simulink model "DFADAS2_SenFus_v1_201204RC_training_210115"  (R2018b)
settings: Solver=FixedStepDiscrete  StartTime=0.0  StopTime=inf  FixedStep=0.002  RelTol=1e-3  EnableMultiTasking=on
PreLoadFcn:
  | RTWConfigurationCB('preloadfcn', bdroot);
libraries: canmsglib x108, simulink x48, canfdmsglib x12
(part 11 of 28)

== system DFADAS2_SenFus_v1_201204RC_training_210115/Signal Input (Input)/Signal Input (10ms) (Input10)/VehInfo/Function Keys State Receive and Processing (FKeyStRx)/Key Enable CAN Frame PreProcess (KeyEnaCANFrmPPrcs) ==
  Bus Creator : BusCreator  Inputs=2
  CAN Diagnosis (CANDia) : Subsystem  Commented=on
  CAN Receive Sample Time : Constant  Value=0.02  OutDataTypeStr=single  SampleTime=-1
  CAN Unpack : canmsglib/CAN Unpack  CANdbFile=F:\LD\3_simulinkModel_13b\TJAHWA\ADAS_D53_PSA1CAN_LiPiao_DLC.dbc  MsgList=GW_309_PSA1  MsgName=GW_309_PSA1  MsgIDType=Standard (11-bit identifier)  MsgIdentifier=777  MsgLength=8  SignalInfo=GW_SCC_LeftSteeringWheelSwitch$0$8$2$2$1$0$1$0$-Inf$Inf$#GW_SCC_RightSteeringWheelSwitch$8$8$2$2$1$0$1$0$-Inf$Inf$#  NSignals=2  IDPort=off  TimestampPort=off  ErrorPort=off  RemotePort=off  LengthPort=off  StatusPort=off  StartBits=str2num('[int32(0);int32(8)]')  SignalSizes=str2num('[int32(8);int32(8)]')  ByteOrders=str2num('[int32(2);int32(2)]')  DataTypes=str2num('[int32(2);int32(2)]')  MultiplexTypes=str2num('[int32(1);int32(1)]')  MultiplexValues=str2num('[double(0);double(0)]')  Factors=str2num('[double(1);double(1)]')  Offsets=str2num('[double(0);double(0)]')  Minimums=str2num('[double(-Inf);double(-Inf)]')  Maximums=str2num('[double(Inf);double(Inf)]')  ApplyMinMax=off
      settings: SourceProductName=Simulink Real-Time  SourceProductBaseCode=XP  DataFormat=CANdb specified signals
  Data Type Conversion1 : DataTypeConversion  OutDataTypeStr=single
  Data Type Conversion3 : DataTypeConversion  OutDataTypeStr=single
  Rate Transition1 : RateTransition  OutPortSampleTime=0.01
  Rate Transition4 : RateTransition  OutPortSampleTime=0.01
  S-Function1 : S-Function  FunctionName=NSTC297CANReceiveBlkLib  Parameters=|  SFunctionDeploymentMode=off  EnableBusSupport=off  mask(NSTC297 CAN Receive){Ns_DeviceID=ADAS Control Unit Gen2, Ns_ChannelNum=4, Ns_FrameID=777, Ns_IsVirtualFrame=off, Ns_RoleInVirtualFrame=Header Frame, Ns_HeaderFrameID=0, Ns_VirtualFrameStatusFlg=off, Ns_IncompleteFrameCntFlg=off, Ns_OverflowCntFlg=off, Ns_FrameBufferSize=1, Ns_SampleTime=0.01}
      | uint16(Ns_DeviceID),
      | uint16(Ns_ChannelNum),
      | uint32(Ns_FrameID),
      | uint8(Ns_IsVirtualFrame),
      | uint16(Ns_RoleInVirtualFrame),
      | uint32(Ns_HeaderFrameID),
      | uint8(Ns_VirtualFrameStatusFlg),
      | uint8(Ns_IncompleteFrameCntFlg),
      | uint8(Ns_OverflowCntFlg),
      | uint16(Ns_FrameBufferSize),
      | double(Ns_SampleTime)
      mask prompts: Ns_DeviceID "Device:"; Ns_ChannelNum "Channel number:"; Ns_FrameID "Frame ID:"; Ns_IsVirtualFrame "Belong to a virtual frame"; Ns_RoleInVirtualFrame "Position in virtual frame:"; Ns_HeaderFrameID "Header frame ID:"; Ns_VirtualFrameStatusFlg "Current virtural frame status output"; Ns_IncompleteFrameCntFlg "Incomplete virtual frame count output"; Ns_OverflowCntFlg "Overflow count output"; Ns_FrameBufferSize "Frame buffer size:"; Ns_SampleTime "Sample time:"
      mask init:
      | NSTC297CANReceive_callback('portlabels');
      mask TypeOptions Ns_DeviceID: General Control Unit Gen2 | ADAS Control Unit Gen2
      mask TypeOptions Ns_ChannelNum: 0 | 1 | 2 | 3 | 4 | 5
      mask Callback Ns_IsVirtualFrame: NSTC297CANReceive_callback('Belong to a virtual frame');
      mask TypeOptions Ns_RoleInVirtualFrame: Header Frame | Data Frame | Trailer Frame
      mask Callback Ns_RoleInVirtualFrame: NSTC297CANReceive_callback('Position in virtual frame');
      mask Display: color('blue');text(0.02,0.9,'NovSteeds TC297','horizontalAlignment','left');color('blue');text(0.5,0.7,'CAN Receive','horizontalAlignment','center');color('black');text(0.5,0.6,'Channel: 4','horizontalAlignment','center');text(0.5,0.5,'ID: 777','horizontalAlignment','center');text(0.5,0.4,'Virtual Frame: No','horizontalAlignment','center');port_label('output',1, 'RemainderCnt');port_label('output',2, 'Msg');
  Time Limit : Constant  OutDataTypeStr=single  SampleTime=-1
  IC_RightSteeringWheelSwitchSig : Outport
  wires:
  Rate Transition4/1 -> Data Type Conversion3/1
  CAN Unpack/1 -> Rate Transition4/1
  CAN Receive Sample Time/1 -> CAN Diagnosis (CANDia)/1(CANDia_tiCANRxSmplT)
  Time Limit/1 -> CAN Diagnosis (CANDia)/2(CANDia_tiTLim)
  S-Function1/1 -> CAN Diagnosis (CANDia)/3(CANDia_cfNewFlg)
  S-Function1/2 -> CAN Unpack/1, CAN Diagnosis (CANDia)/4(CANDia_regCANMsg)
  Rate Transition1/1 -> Data Type Conversion1/1
  CAN Unpack/2 -> Rate Transition1/1
  Data Type Conversion3/1 -> Bus Creator/1  "GW_LeftSteeringWheelS"
  Data Type Conversion1/1 -> Bus Creator/2  "GW_RightSteeringWheelS"
  Bus Creator/1 -> IC_RightSteeringWheelSwitchSig/1

== system DFADAS2_SenFus_v1_201204RC_training_210115/Signal Input (Input)/Signal Input (10ms) (Input10)/VehInfo/MP5 Signal Receive (MP5Rx)1/CAN Diagnosis (CANDia) ==
  CANDia_tiCANRxSmplT : Inport
  CANDia_tiTLim : Inport  Port=2
  CANDia_cfNewFlg : Inport  Port=3
  CANDia_regCANMsg : Inport  Port=4
  CANDia_ctRllCnt : Inport  Port=5
  Break State Diagnosis (BreStDia) : Subsystem
  CAN Frame DTC Generator (CANFrmDTCGtr) : Subsystem
  CheckSum Diagnosis (ChkSumDia) : Subsystem
  RollingCounter Diagnosis (RllCntDia) : Subsystem
  wires:
  CANDia_regCANMsg/1 -> CheckSum Diagnosis (ChkSumDia)/1(ChkSumDia_regCANMsgPrev)
  CANDia_ctRllCnt/1 -> RollingCounter Diagnosis (RllCntDia)/1(RllCntChk_ctRollingCounter)
  RollingCounter Diagnosis (RllCntDia)/1(RllCntChk_efErrorFlag) -> CAN Frame DTC Generator (CANFrmDTCGtr)/3(CANFrmDTCGtr_efRllCntDiaErrFlg)
  Break State Diagnosis (BreStDia)/1(BreStDia_efErrFlg) -> CAN Frame DTC Generator (CANFrmDTCGtr)/1(CANFrmDTCGtr_efBreStDiaErrFlg)
  CheckSum Diagnosis (ChkSumDia)/1(ChkSumDia_efErrFlg) -> CAN Frame DTC Generator (CANFrmDTCGtr)/2(CANFrmDTCGtr_efChkSumDiaErrFlg)
  CANDia_cfNewFlg/1 -> Break State Diagnosis (BreStDia)/3(BreStDia_cfCANRxNewFlg)
  CANDia_tiTLim/1 -> Break State Diagnosis (BreStDia)/2(BreStDia_tiTLim)
  CANDia_tiCANRxSmplT/1 -> Break State Diagnosis (BreStDia)/1(BreStDia_tiCANRxSmplT)

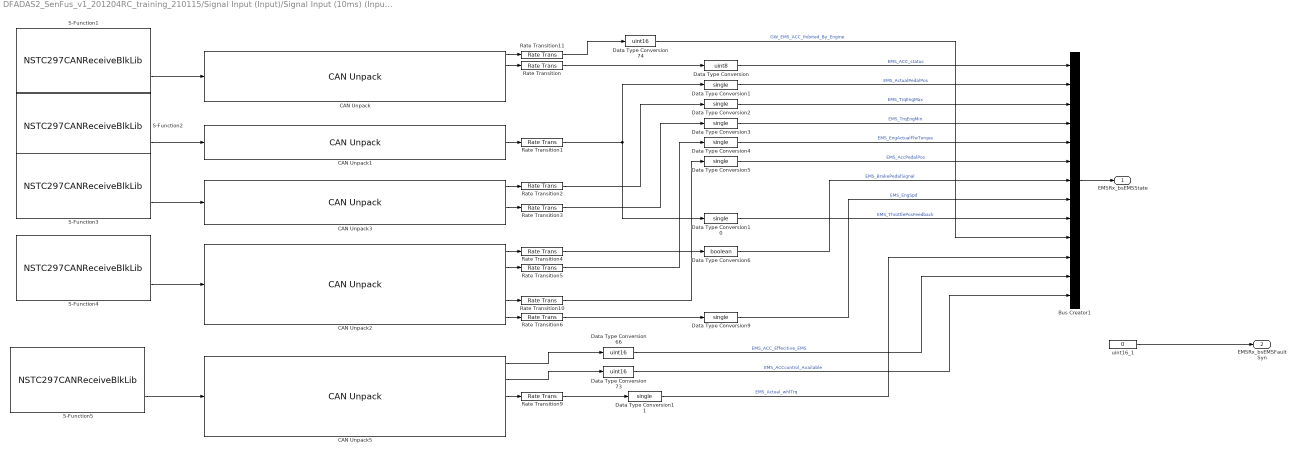
== system DFADAS2_SenFus_v1_201204RC_training_210115/Signal Input (Input)/Signal Input (10ms) (Input10)/VehInfo/Powertrain State Receive and Processing (PTRx)/EMS State Receive and Processing (EMSRx) ==
  Bus Creator1 : BusCreator  Inputs=13
  CAN Unpack : canmsglib/CAN Unpack  CANdbFile=F:\ADAS_File\ACC_AEB_D53_20190520\ADAS_ECU_PSA1_CAN_V2_v20190520.dbc  MsgList=GW_2D8_PSA1  MsgName=GW_2D8_PSA1  MsgIDType=Standard (11-bit identifier)  MsgIdentifier=728  MsgLength=7  SignalInfo=GW_EMS_ACC_Ihibited_By_Engine$52$1$2$2$1$0$1$0$0$1$#GW_EMS_EMS_Status_ACC$16$3$2$2$1$0$1$0$0$7$#GW_EMS_Pot_WhlTrq_Max$37$11$2$2$1$0$8$-4000$-4000$11000$#GW_EMS_Pot_WhlTrq_Min$53$11$2$2$1$0$8$-4000$-4000$11000$#GW_EMS_Pot_WhlTrq_Request$19$13$2$2$1$0$2$-4000$-4000$11000$#  NSignals=5  IDPort=off  TimestampPort=off  ErrorPort=off  RemotePort=off  LengthPort=off  StatusPort=off  StartBits=str2num('[int32(52);int32(16);int32(37);int32(53);int32(19)]')  SignalSizes=str2num('[int32(1);int32(3);int32(11);int32(11);int32(13)]')  ByteOrders=str2num('[int32(2);int32(2);int32(2);int32(2);int32(2)]')  DataTypes=str2num('[int32(2);int32(2);int32(2);int32(2);int32(2)]')  MultiplexTypes=str2num('[int32(1);int32(1);int32(1);int32(1);int32(1)]')  MultiplexValues=str2num('[double(0);double(0);double(0);double(0);double(0)]')  Factors=str2num('[double(1);double(1);double(8);double(8);double(2)]')  Offsets=str2num('[double(0);double(0);double(-4000);double(-4000);double(-4000)]')  Minimums=str2num('[double(0);double(0);double(-4000);double(-4000);double(-4000)]')  Maximums=str2num('[double(1);double(7);double(11000);double(11000);double(11000)]')  ApplyMinMax=off
      settings: SourceProductName=Simulink Real-Time  SourceProductBaseCode=XP  DataFormat=CANdb specified signals
  CAN Unpack1 : canmsglib/CAN Unpack  CANdbFile=F:\ADAS_File\ACC_AEB_D53_20190520\ADAS_ECU_PSA1_CAN_V2_v20190520.dbc  MsgList=GW_228_PSA1  MsgName=GW_228_PSA1  MsgIDType=Standard (11-bit identifier)  MsgIdentifier=552  MsgLength=8  SignalInfo=EMS_Acceleration_pedal_position$16$8$2$2$1$0$5.000000e-01$0$0$100$#  NSignals=1  IDPort=off  TimestampPort=off  ErrorPort=off  RemotePort=off  LengthPort=off  StatusPort=off  StartBits=str2num('[int32(16)]')  SignalSizes=str2num('[int32(8)]')  ByteOrders=str2num('[int32(2)]')  DataTypes=str2num('[int32(2)]')  MultiplexTypes=str2num('[int32(1)]')  MultiplexValues=str2num('[double(0)]')  Factors=str2num('[double(5.000000e-01)]')  Offsets=str2num('[double(0)]')  Minimums=str2num('[double(0)]')  Maximums=str2num('[double(100)]')  ApplyMinMax=off
      settings: SourceProductName=Simulink Real-Time  SourceProductBaseCode=XP  DataFormat=CANdb specified signals
  CAN Unpack2 : canmsglib/CAN Unpack  CANdbFile=F:\ADAS_File\ACC_AEB_D53_20190520\ADAS_ECU_PSA1_CAN_V2_v20190520.dbc  MsgList=GW_208_PSA1  MsgName=GW_208_PSA1  MsgIDType=Standard (11-bit identifier)  MsgIdentifier=520  MsgLength=8  SignalInfo=Brake_secondary_contact$33$1$2$2$1$0$1$0$-Inf$Inf$#EMS_Actual_torque$16$8$2$2$1$0$2$-100$-100$408$#EMS_DiagMuxOn$38$1$2$2$1$0$1$0$-Inf$Inf$#EMS_Driver_request$24$8$2$2$1$0$5.000000e-01$0$0$100$#EMS_Engine_RPM$8$16$2$2$1$0$1.250000e-01$0$0$8.191750e+03$#  NSignals=5  IDPort=off  TimestampPort=off  ErrorPort=off  RemotePort=off  LengthPort=off  StatusPort=off  StartBits=str2num('[int32(33);int32(16);int32(38);int32(24);int32(8)]')  SignalSizes=str2num('[int32(1);int32(8);int32(1);int32(8);int32(16)]')  ByteOrders=str2num('[int32(2);int32(2);int32(2);int32(2);int32(2)]')  DataTypes=str2num('[int32(2);int32(2);int32(2);int32(2);int32(2)]')  MultiplexTypes=str2num('[int32(1);int32(1);int32(1);int32(1);int32(1)]')  MultiplexValues=str2num('[double(0);double(0);double(0);double(0);double(0)]')  Factors=str2num('[double(1);double(2);double(1);double(5.000000e-01);double(1.250000e-01)]')  Offsets=str2num('[double(0);double(-100);double(0);double(0);double(0)]')  Minimums=str2num('[double(-Inf);double(-100);double(-Inf);double(0);double(0)]')  Maximums=str2num('[double(Inf);double(408);double(Inf);double(100);double(8.191750e+03)]')  ApplyMinMax=off
      settings: SourceProductName=Simulink Real-Time  SourceProductBaseCode=XP  DataFormat=CANdb specified signals
  CAN Unpack3 : canmsglib/CAN Unpack  CANdbFile=F:\ADAS_File\ACC_AEB_D53_20190520\ADAS_ECU_PSA1_CAN_V2_v20190520.dbc  MsgList=GW_2F8_PSA1  MsgName=GW_2F8_PSA1  MsgIDType=Standard (11-bit identifier)  MsgIdentifier=760  MsgLength=7  SignalInfo=EMS_WhlTrq_max$19$13$2$2$1$0$2$-4000$-4000$11000$#EMS_WhlTrq_max_offset$24$11$2$2$1$0$2$0$0$4000$#EMS_WhlTrq_min$43$13$2$2$1$0$2$-4000$-4000$11000$#EMS_WhlTrq_min_offset$48$11$2$2$1$0$2$0$0$4000$#  NSignals=4  IDPort=off  TimestampPort=off  ErrorPort=off  RemotePort=off  LengthPort=off  StatusPort=off  StartBits=str2num('[int32(19);int32(24);int32(43);int32(48)]')  SignalSizes=str2num('[int32(13);int32(11);int32(13);int32(11)]')  ByteOrders=str2num('[int32(2);int32(2);int32(2);int32(2)]')  DataTypes=str2num('[int32(2);int32(2);int32(2);int32(2)]')  MultiplexTypes=str2num('[int32(1);int32(1);int32(1);int32(1)]')  MultiplexValues=str2num('[double(0);double(0);double(0);double(0)]')  Factors=str2num('[double(2);double(2);double(2);double(2)]')  Offsets=str2num('[double(-4000);double(0);double(-4000);double(0)]')  Minimums=str2num('[double(-4000);double(0);double(-4000);double(0)]')  Maximums=str2num('[double(11000);double(4000);double(11000);double(4000)]')  ApplyMinMax=off
      settings: SourceProductName=Simulink Real-Time  SourceProductBaseCode=XP  DataFormat=CANdb specified signals
  CAN Unpack5 : canmsglib/CAN Unpack  CANdbFile=F:\ADAS_File\ACC_AEB_D53_20190520\ADAS_ECU_PSA1_CAN_V2_v20190520.dbc  MsgList=GW_318_PSA1  MsgName=GW_318_PSA1  MsgIDType=Standard (11-bit identifier)  MsgIdentifier=792  MsgLength=5  SignalInfo=EMS_ACC_Effecitive_EMS$33$1$2$2$1$0$1$0$0$1$#EMS_ACCcontrol_Available$17$1$2$2$1$0$1$0$0$1$#EMS_Actual_whlTrq$34$14$2$2$1$0$1$-4000$-4000$11000$#EMS_Driver_wheel_torque$18$14$2$2$1$0$1$-4000$-4000$11000$#EMS_GearBox_ACCcontrol_Available$16$1$2$2$1$0$1$0$0$1$#  NSignals=5  IDPort=off  TimestampPort=off  ErrorPort=off  RemotePort=off  LengthPort=off  StatusPort=off  StartBits=str2num('[int32(33);int32(17);int32(34);int32(18);int32(16)]')  SignalSizes=str2num('[int32(1);int32(1);int32(14);int32(14);int32(1)]')  ByteOrders=str2num('[int32(2);int32(2);int32(2);int32(2);int32(2)]')  DataTypes=str2num('[int32(2);int32(2);int32(2);int32(2);int32(2)]')  MultiplexTypes=str2num('[int32(1);int32(1);int32(1);int32(1);int32(1)]')  MultiplexValues=str2num('[double(0);double(0);double(0);double(0);double(0)]')  Factors=str2num('[double(1);double(1);double(1);double(1);double(1)]')  Offsets=str2num('[double(0);double(0);double(-4000);double(-4000);double(0)]')  Minimums=str2num('[double(0);double(0);double(-4000);double(-4000);double(0)]')  Maximums=str2num('[double(1);double(1);double(11000);double(11000);double(1)]')  ApplyMinMax=off
      settings: SourceProductName=Simulink Real-Time  SourceProductBaseCode=XP  DataFormat=CANdb specified signals
  Data Type Conversion : DataTypeConversion  OutDataTypeStr=uint8
  Data Type Conversion{1..5,9..11} (8 alike) : DataTypeConversion  OutDataTypeStr=single
  Data Type Conversion6 : DataTypeConversion  OutDataTypeStr=boolean
  Data Type Conversion66 : DataTypeConversion  OutDataTypeStr=uint16
  Data Type Conversion73 : DataTypeConversion  OutDataTypeStr=uint16
  Data Type Conversion74 : DataTypeConversion  OutDataTypeStr=uint16
  Rate Transition{,1..6,9..11} (10 alike) : RateTransition  OutPortSampleTime=0.01
  S-Function1 : S-Function  FunctionName=NSTC297CANReceiveBlkLib  Parameters=|  SFunctionDeploymentMode=off  EnableBusSupport=off  mask(NSTC297 CAN Receive){Ns_DeviceID=ADAS Control Unit Gen2, Ns_ChannelNum=4, Ns_FrameID=728, Ns_IsVirtualFrame=off, Ns_RoleInVirtualFrame=Header Frame, Ns_HeaderFrameID=0, Ns_VirtualFrameStatusFlg=off, Ns_IncompleteFrameCntFlg=off, Ns_OverflowCntFlg=off, Ns_FrameBufferSize=1, Ns_SampleTime=0.02}
      | uint16(Ns_DeviceID),
      | uint16(Ns_ChannelNum),
      | uint32(Ns_FrameID),
      | uint8(Ns_IsVirtualFrame),
      | uint16(Ns_RoleInVirtualFrame),
      | uint32(Ns_HeaderFrameID),
      | uint8(Ns_VirtualFrameStatusFlg),
      | uint8(Ns_IncompleteFrameCntFlg),
      | uint8(Ns_OverflowCntFlg),
      | uint16(Ns_FrameBufferSize),
      | double(Ns_SampleTime)
      mask prompts: Ns_DeviceID "Device:"; Ns_ChannelNum "Channel number:"; Ns_FrameID "Frame ID:"; Ns_IsVirtualFrame "Belong to a virtual frame"; Ns_RoleInVirtualFrame "Position in virtual frame:"; Ns_HeaderFrameID "Header frame ID:"; Ns_VirtualFrameStatusFlg "Current virtural frame status output"; Ns_IncompleteFrameCntFlg "Incomplete virtual frame count output"; Ns_OverflowCntFlg "Overflow count output"; Ns_FrameBufferSize "Frame buffer size:"; Ns_SampleTime "Sample time:"
      mask init:
      | NSTC297CANReceive_callback('portlabels');
      mask TypeOptions Ns_DeviceID: General Control Unit Gen2 | ADAS Control Unit Gen2
      mask TypeOptions Ns_ChannelNum: 0 | 1 | 2 | 3 | 4 | 5
      mask Callback Ns_IsVirtualFrame: NSTC297CANReceive_callback('Belong to a virtual frame');
      mask TypeOptions Ns_RoleInVirtualFrame: Header Frame | Data Frame | Trailer Frame
      mask Callback Ns_RoleInVirtualFrame: NSTC297CANReceive_callback('Position in virtual frame');
      mask Display: color('blue');text(0.02,0.9,'NovSteeds TC297','horizontalAlignment','left');color('blue');text(0.5,0.7,'CAN Receive','horizontalAlignment','center');color('black');text(0.5,0.6,'Channel: 4','horizontalAlignment','center');text(0.5,0.5,'ID: 728','horizontalAlignment','center');text(0.5,0.4,'Virtual Frame: No','horizontalAlignment','center');port_label('output',1, 'RemainderCnt');port_label('output',2, 'Msg');
  S-Function2 : S-Function  FunctionName=NSTC297CANReceiveBlkLib  Parameters=|  SFunctionDeploymentMode=off  EnableBusSupport=off  mask(NSTC297 CAN Receive){Ns_DeviceID=ADAS Control Unit Gen2, Ns_ChannelNum=4, Ns_FrameID=552, Ns_IsVirtualFrame=off, Ns_RoleInVirtualFrame=Header Frame, Ns_HeaderFrameID=0, Ns_VirtualFrameStatusFlg=off, Ns_IncompleteFrameCntFlg=off, Ns_OverflowCntFlg=off, Ns_FrameBufferSize=1, Ns_SampleTime=0.01}
      | uint16(Ns_DeviceID),
      | uint16(Ns_ChannelNum),
      | uint32(Ns_FrameID),
      | uint8(Ns_IsVirtualFrame),
      | uint16(Ns_RoleInVirtualFrame),
      | uint32(Ns_HeaderFrameID),
      | uint8(Ns_VirtualFrameStatusFlg),
      | uint8(Ns_IncompleteFrameCntFlg),
      | uint8(Ns_OverflowCntFlg),
      | uint16(Ns_FrameBufferSize),
      | double(Ns_SampleTime)
      mask prompts: Ns_DeviceID "Device:"; Ns_ChannelNum "Channel number:"; Ns_FrameID "Frame ID:"; Ns_IsVirtualFrame "Belong to a virtual frame"; Ns_RoleInVirtualFrame "Position in virtual frame:"; Ns_HeaderFrameID "Header frame ID:"; Ns_VirtualFrameStatusFlg "Current virtural frame status output"; Ns_IncompleteFrameCntFlg "Incomplete virtual frame count output"; Ns_OverflowCntFlg "Overflow count output"; Ns_FrameBufferSize "Frame buffer size:"; Ns_SampleTime "Sample time:"
      mask init:
      | NSTC297CANReceive_callback('portlabels');
      mask TypeOptions Ns_DeviceID: General Control Unit Gen2 | ADAS Control Unit Gen2
      mask TypeOptions Ns_ChannelNum: 0 | 1 | 2 | 3 | 4 | 5
      mask Callback Ns_IsVirtualFrame: NSTC297CANReceive_callback('Belong to a virtual frame');
      mask TypeOptions Ns_RoleInVirtualFrame: Header Frame | Data Frame | Trailer Frame
      mask Callback Ns_RoleInVirtualFrame: NSTC297CANReceive_callback('Position in virtual frame');
      mask Display: color('blue');text(0.02,0.9,'NovSteeds TC297','horizontalAlignment','left');color('blue');text(0.5,0.7,'CAN Receive','horizontalAlignment','center');color('black');text(0.5,0.6,'Channel: 4','horizontalAlignment','center');text(0.5,0.5,'ID: 552','horizontalAlignment','center');text(0.5,0.4,'Virtual Frame: No','horizontalAlignment','center');port_label('output',1, 'RemainderCnt');port_label('output',2, 'Msg');
  S-Function3 : S-Function  FunctionName=NSTC297CANReceiveBlkLib  Parameters=|  SFunctionDeploymentMode=off  EnableBusSupport=off  mask(NSTC297 CAN Receive){Ns_DeviceID=ADAS Control Unit Gen2, Ns_ChannelNum=4, Ns_FrameID=760, Ns_IsVirtualFrame=off, Ns_RoleInVirtualFrame=Header Frame, Ns_HeaderFrameID=0, Ns_VirtualFrameStatusFlg=off, Ns_IncompleteFrameCntFlg=off, Ns_OverflowCntFlg=off, Ns_FrameBufferSize=1, Ns_SampleTime=0.02}
      | uint16(Ns_DeviceID),
      | uint16(Ns_ChannelNum),
      | uint32(Ns_FrameID),
      | uint8(Ns_IsVirtualFrame),
      | uint16(Ns_RoleInVirtualFrame),
      | uint32(Ns_HeaderFrameID),
      | uint8(Ns_VirtualFrameStatusFlg),
      | uint8(Ns_IncompleteFrameCntFlg),
      | uint8(Ns_OverflowCntFlg),
      | uint16(Ns_FrameBufferSize),
      | double(Ns_SampleTime)
      mask prompts: Ns_DeviceID "Device:"; Ns_ChannelNum "Channel number:"; Ns_FrameID "Frame ID:"; Ns_IsVirtualFrame "Belong to a virtual frame"; Ns_RoleInVirtualFrame "Position in virtual frame:"; Ns_HeaderFrameID "Header frame ID:"; Ns_VirtualFrameStatusFlg "Current virtural frame status output"; Ns_IncompleteFrameCntFlg "Incomplete virtual frame count output"; Ns_OverflowCntFlg "Overflow count output"; Ns_FrameBufferSize "Frame buffer size:"; Ns_SampleTime "Sample time:"
      mask init:
      | NSTC297CANReceive_callback('portlabels');
      mask TypeOptions Ns_DeviceID: General Control Unit Gen2 | ADAS Control Unit Gen2
      mask TypeOptions Ns_ChannelNum: 0 | 1 | 2 | 3 | 4 | 5
      mask Callback Ns_IsVirtualFrame: NSTC297CANReceive_callback('Belong to a virtual frame');
      mask TypeOptions Ns_RoleInVirtualFrame: Header Frame | Data Frame | Trailer Frame
      mask Callback Ns_RoleInVirtualFrame: NSTC297CANReceive_callback('Position in virtual frame');
      mask Display: color('blue');text(0.02,0.9,'NovSteeds TC297','horizontalAlignment','left');color('blue');text(0.5,0.7,'CAN Receive','horizontalAlignment','center');color('black');text(0.5,0.6,'Channel: 4','horizontalAlignment','center');text(0.5,0.5,'ID: 760','horizontalAlignment','center');text(0.5,0.4,'Virtual Frame: No','horizontalAlignment','center');port_label('output',1, 'RemainderCnt');port_label('output',2, 'Msg');
  S-Function4 : S-Function  FunctionName=NSTC297CANReceiveBlkLib  Parameters=|  SFunctionDeploymentMode=off  EnableBusSupport=off  mask(NSTC297 CAN Receive){Ns_DeviceID=ADAS Control Unit Gen2, Ns_ChannelNum=4, Ns_FrameID=520, Ns_IsVirtualFrame=off, Ns_RoleInVirtualFrame=Header Frame, Ns_HeaderFrameID=0, Ns_VirtualFrameStatusFlg=off, Ns_IncompleteFrameCntFlg=off, Ns_OverflowCntFlg=off, Ns_FrameBufferSize=1, Ns_SampleTime=0.01}
      | uint16(Ns_DeviceID),
      | uint16(Ns_ChannelNum),
      | uint32(Ns_FrameID),
      | uint8(Ns_IsVirtualFrame),
      | uint16(Ns_RoleInVirtualFrame),
      | uint32(Ns_HeaderFrameID),
      | uint8(Ns_VirtualFrameStatusFlg),
      | uint8(Ns_IncompleteFrameCntFlg),
      | uint8(Ns_OverflowCntFlg),
      | uint16(Ns_FrameBufferSize),
      | double(Ns_SampleTime)
      mask prompts: Ns_DeviceID "Device:"; Ns_ChannelNum "Channel number:"; Ns_FrameID "Frame ID:"; Ns_IsVirtualFrame "Belong to a virtual frame"; Ns_RoleInVirtualFrame "Position in virtual frame:"; Ns_HeaderFrameID "Header frame ID:"; Ns_VirtualFrameStatusFlg "Current virtural frame status output"; Ns_IncompleteFrameCntFlg "Incomplete virtual frame count output"; Ns_OverflowCntFlg "Overflow count output"; Ns_FrameBufferSize "Frame buffer size:"; Ns_SampleTime "Sample time:"
      mask init:
      | NSTC297CANReceive_callback('portlabels');
      mask TypeOptions Ns_DeviceID: General Control Unit Gen2 | ADAS Control Unit Gen2
      mask TypeOptions Ns_ChannelNum: 0 | 1 | 2 | 3 | 4 | 5
      mask Callback Ns_IsVirtualFrame: NSTC297CANReceive_callback('Belong to a virtual frame');
      mask TypeOptions Ns_RoleInVirtualFrame: Header Frame | Data Frame | Trailer Frame
      mask Callback Ns_RoleInVirtualFrame: NSTC297CANReceive_callback('Position in virtual frame');
      mask Display: color('blue');text(0.02,0.9,'NovSteeds TC297','horizontalAlignment','left');color('blue');text(0.5,0.7,'CAN Receive','horizontalAlignment','center');color('black');text(0.5,0.6,'Channel: 4','horizontalAlignment','center');text(0.5,0.5,'ID: 520','horizontalAlignment','center');text(0.5,0.4,'Virtual Frame: No','horizontalAlignment','center');port_label('output',1, 'RemainderCnt');port_label('output',2, 'Msg');
  S-Function5 : S-Function  FunctionName=NSTC297CANReceiveBlkLib  Parameters=|  SFunctionDeploymentMode=off  EnableBusSupport=off  mask(NSTC297 CAN Receive){Ns_DeviceID=ADAS Control Unit Gen2, Ns_ChannelNum=4, Ns_FrameID=792, Ns_IsVirtualFrame=off, Ns_RoleInVirtualFrame=Header Frame, Ns_HeaderFrameID=0, Ns_VirtualFrameStatusFlg=off, Ns_IncompleteFrameCntFlg=off, Ns_OverflowCntFlg=off, Ns_FrameBufferSize=1, Ns_SampleTime=0.01}
      | uint16(Ns_DeviceID),
      | uint16(Ns_ChannelNum),
      | uint32(Ns_FrameID),
      | uint8(Ns_IsVirtualFrame),
      | uint16(Ns_RoleInVirtualFrame),
      | uint32(Ns_HeaderFrameID),
      | uint8(Ns_VirtualFrameStatusFlg),
      | uint8(Ns_IncompleteFrameCntFlg),
      | uint8(Ns_OverflowCntFlg),
      | uint16(Ns_FrameBufferSize),
      | double(Ns_SampleTime)
      mask prompts: Ns_DeviceID "Device:"; Ns_ChannelNum "Channel number:"; Ns_FrameID "Frame ID:"; Ns_IsVirtualFrame "Belong to a virtual frame"; Ns_RoleInVirtualFrame "Position in virtual frame:"; Ns_HeaderFrameID "Header frame ID:"; Ns_VirtualFrameStatusFlg "Current virtural frame status output"; Ns_IncompleteFrameCntFlg "Incomplete virtual frame count output"; Ns_OverflowCntFlg "Overflow count output"; Ns_FrameBufferSize "Frame buffer size:"; Ns_SampleTime "Sample time:"
      mask init:
      | NSTC297CANReceive_callback('portlabels');
      mask TypeOptions Ns_DeviceID: General Control Unit Gen2 | ADAS Control Unit Gen2
      mask TypeOptions Ns_ChannelNum: 0 | 1 | 2 | 3 | 4 | 5
      mask Callback Ns_IsVirtualFrame: NSTC297CANReceive_callback('Belong to a virtual frame');
      mask TypeOptions Ns_RoleInVirtualFrame: Header Frame | Data Frame | Trailer Frame
      mask Callback Ns_RoleInVirtualFrame: NSTC297CANReceive_callback('Position in virtual frame');
      mask Display: color('blue');text(0.02,0.9,'NovSteeds TC297','horizontalAlignment','left');color('blue');text(0.5,0.7,'CAN Receive','horizontalAlignment','center');color('black');text(0.5,0.6,'Channel: 4','horizontalAlignment','center');text(0.5,0.5,'ID: 792','horizontalAlignment','center');text(0.5,0.4,'Virtual Frame: No','horizontalAlignment','center');port_label('output',1, 'RemainderCnt');port_label('output',2, 'Msg');
  uint16_1 : Constant  Value=0  OutDataTypeStr=uint16
  EMSRx_bsEMSState : Outport
  EMSRx_bsEMSFaultSyn : Outport  Port=2
  wires:
  uint16_1/1 -> EMSRx_bsEMSFaultSyn/1
  Bus Creator1/1 -> EMSRx_bsEMSState/1
  CAN Unpack2/2 -> Rate Transition5/1
  CAN Unpack/2 -> Rate Transition/1
  CAN Unpack3/1 -> Rate Transition2/1
  CAN Unpack3/3 -> Rate Transition3/1
  CAN Unpack2/1 -> Rate Transition4/1
  CAN Unpack2/5 -> Rate Transition6/1
  CAN Unpack1/1 -> Rate Transition1/1
  Data Type Conversion/1 -> Bus Creator1/1  "EMS_ACC_status"
  Data Type Conversion1/1 -> Bus Creator1/2  "EMS_ActualPedalPos"
  Data Type Conversion2/1 -> Bus Creator1/3  "EMS_TrqEngMax"
  Data Type Conversion3/1 -> Bus Creator1/4  "EMS_TrqEngMin"
  Data Type Conversion4/1 -> Bus Creator1/5  "EMS_EngActualFlwTorque"
  Data Type Conversion5/1 -> Bus Creator1/6  "EMS_AccPedalPos"
  Data Type Conversion6/1 -> Bus Creator1/7  "EMS_BrakePedalSignal"
  Data Type Conversion9/1 -> Bus Creator1/8  "EMS_EngSpd"
  Data Type Conversion10/1 -> Bus Creator1/9  "EMS_ThrottlePosFeedback"
  S-Function2/2 -> CAN Unpack1/1
  S-Function1/2 -> CAN Unpack/1
  S-Function4/2 -> CAN Unpack2/1
  S-Function3/2 -> CAN Unpack3/1
  Rate Transition/1 -> Data Type Conversion/1
  Rate Transition1/1 -> Data Type Conversion10/1, Data Type Conversion1/1
  Rate Transition2/1 -> Data Type Conversion2/1
  Rate Transition3/1 -> Data Type Conversion3/1
  Rate Transition4/1 -> Data Type Conversion6/1
  Rate Transition5/1 -> Data Type Conversion4/1
  Rate Transition6/1 -> Data Type Conversion9/1
  S-Function5/2 -> CAN Unpack5/1
  CAN Unpack5/3 -> Rate Transition9/1
  Rate Transition9/1 -> Data Type Conversion11/1
  Data Type Conversion11/1 -> Bus Creator1/11  "EMS_Actual_whlTrq"
  CAN Unpack2/4 -> Rate Transition10/1
  Rate Transition10/1 -> Data Type Conversion5/1
  Data Type Conversion66/1 -> Bus Creator1/12  "EMS_ACC_Effecitive_EMS"
  Data Type Conversion74/1 -> Bus Creator1/10  "GW_EMS_ACC_Ihibited_By_Engine"
  Data Type Conversion73/1 -> Bus Creator1/13  "EMS_ACCcontrol_Available"
  CAN Unpack5/1 -> Data Type Conversion66/1
  CAN Unpack5/2 -> Data Type Conversion73/1
  CAN Unpack/1 -> Rate Transition11/1
  Rate Transition11/1 -> Data Type Conversion74/1

== system DFADAS2_SenFus_v1_201204RC_training_210115/Signal Input (Input)/Signal Input (10ms) (Input10)/VehInfo/Powertrain State Receive and Processing (PTRx)/TCU State Receive and Processing (TCURx) ==
  Bus Creator1 : BusCreator  Inputs=2
  CAN Unpack6 : canmsglib/CAN Unpack  CANdbFile=F:\ADAS_File\ACC_AEB_D53_20190520\ADAS_ECU_PSA1_CAN_V2_v20190520.dbc  MsgList=GW_349_PSA1  MsgName=GW_349_PSA1  MsgIDType=Standard (11-bit identifier)  MsgIdentifier=841  MsgLength=8  SignalInfo=BV_dynamic_frame_checksum$52$4$2$2$1$0$1$0$-Inf$Inf$#TCU_AGB_Target_position$28$4$2$2$1$0$1$0$-Inf$Inf$#TCU_Gear_lever_position$24$4$2$2$1$0$1$0$-Inf$Inf$#bits_Compute_for_Gear_Box$48$4$2$2$1$0$1$0$0$15$#  NSignals=4  IDPort=off  TimestampPort=off  ErrorPort=off  RemotePort=off  LengthPort=off  StatusPort=off  StartBits=str2num('[int32(52);int32(28);int32(24);int32(48)]')  SignalSizes=str2num('[int32(4);int32(4);int32(4);int32(4)]')  ByteOrders=str2num('[int32(2);int32(2);int32(2);int32(2)]')  DataTypes=str2num('[int32(2);int32(2);int32(2);int32(2)]')  MultiplexTypes=str2num('[int32(1);int32(1);int32(1);int32(1)]')  MultiplexValues=str2num('[double(0);double(0);double(0);double(0)]')  Factors=str2num('[double(1);double(1);double(1);double(1)]')  Offsets=str2num('[double(0);double(0);double(0);double(0)]')  Minimums=str2num('[double(-Inf);double(-Inf);double(-Inf);double(0)]')  Maximums=str2num('[double(Inf);double(Inf);double(Inf);double(15)]')  ApplyMinMax=off
      settings: SourceProductName=Simulink Real-Time  SourceProductBaseCode=XP  DataFormat=CANdb specified signals
  Data Type Conversion7 : DataTypeConversion  OutDataTypeStr=uint8
  Data Type Conversion8 : DataTypeConversion  OutDataTypeStr=uint8
  S-Function1 : S-Function  FunctionName=NSTC297CANReceiveBlkLib  Parameters=|  SFunctionDeploymentMode=off  EnableBusSupport=off  mask(NSTC297 CAN Receive){Ns_DeviceID=ADAS Control Unit Gen2, Ns_ChannelNum=4, Ns_FrameID=841, Ns_IsVirtualFrame=off, Ns_RoleInVirtualFrame=Header Frame, Ns_HeaderFrameID=0, Ns_VirtualFrameStatusFlg=off, Ns_IncompleteFrameCntFlg=off, Ns_OverflowCntFlg=off, Ns_FrameBufferSize=1, Ns_SampleTime=0.01}
      | uint16(Ns_DeviceID),
      | uint16(Ns_ChannelNum),
      | uint32(Ns_FrameID),
      | uint8(Ns_IsVirtualFrame),
      | uint16(Ns_RoleInVirtualFrame),
      | uint32(Ns_HeaderFrameID),
      | uint8(Ns_VirtualFrameStatusFlg),
      | uint8(Ns_IncompleteFrameCntFlg),
      | uint8(Ns_OverflowCntFlg),
      | uint16(Ns_FrameBufferSize),
      | double(Ns_SampleTime)
      mask prompts: Ns_DeviceID "Device:"; Ns_ChannelNum "Channel number:"; Ns_FrameID "Frame ID:"; Ns_IsVirtualFrame "Belong to a virtual frame"; Ns_RoleInVirtualFrame "Position in virtual frame:"; Ns_HeaderFrameID "Header frame ID:"; Ns_VirtualFrameStatusFlg "Current virtural frame status output"; Ns_IncompleteFrameCntFlg "Incomplete virtual frame count output"; Ns_OverflowCntFlg "Overflow count output"; Ns_FrameBufferSize "Frame buffer size:"; Ns_SampleTime "Sample time:"
      mask init:
      | NSTC297CANReceive_callback('portlabels');
      mask TypeOptions Ns_DeviceID: General Control Unit Gen2 | ADAS Control Unit Gen2
      mask TypeOptions Ns_ChannelNum: 0 | 1 | 2 | 3 | 4 | 5
      mask Callback Ns_IsVirtualFrame: NSTC297CANReceive_callback('Belong to a virtual frame');
      mask TypeOptions Ns_RoleInVirtualFrame: Header Frame | Data Frame | Trailer Frame
      mask Callback Ns_RoleInVirtualFrame: NSTC297CANReceive_callback('Position in virtual frame');
      mask Display: color('blue');text(0.02,0.9,'NovSteeds TC297','horizontalAlignment','left');color('blue');text(0.5,0.7,'CAN Receive','horizontalAlignment','center');color('black');text(0.5,0.6,'Channel: 4','horizontalAlignment','center');text(0.5,0.5,'ID: 841','horizontalAlignment','center');text(0.5,0.4,'Virtual Frame: No','horizontalAlignment','center');port_label('output',1, 'RemainderCnt');port_label('output',2, 'Msg');
  uint16_1 : Constant  Value=0  OutDataTypeStr=uint16
  TCURx_bsTCUState : Outport
  TCURx_bsTCUFaultSyn : Outport  Port=2
  wires:
  uint16_1/1 -> TCURx_bsTCUFaultSyn/1
  CAN Unpack6/2 -> Data Type Conversion8/1
  CAN Unpack6/3 -> Data Type Conversion7/1
  Data Type Conversion7/1 -> Bus Creator1/2  "TCU_ActualGear"
  Data Type Conversion8/1 -> Bus Creator1/1  "TCU_TargetGear"
  S-Function1/2 -> CAN Unpack6/1
  Bus Creator1/1 -> TCURx_bsTCUState/1

== system DFADAS2_SenFus_v1_201204RC_training_210115/Signal Input (Input)/Signal Input (10ms) (Input10)/VehInfo/Vehicle Movement Signal Receive and Processing (VehMovRx)/Fault Synthesis (FaultSyn) ==
  in1 : Inport
  in2 : Inport  Port=2
  in3 : Inport  Port=3
  in4 : Inport  Port=4
  in5 : Inport  Port=5
  FaultSyn_efFaultSyn : Outport

== system DFADAS2_SenFus_v1_201204RC_training_210115/Signal Input (Input)/Signal Input (10ms) (Input10)/VehInfo/Vehicle Movement Signal Receive and Processing (VehMovRx)/Fault Synthesis (FaultSyn)1 ==
  in1 : Inport
  in2 : Inport  Port=2
  in3 : Inport  Port=3
  in4 : Inport  Port=4
  in5 : Inport  Port=5
  in6 : Inport  Port=6
  in7 : Inport  Port=7
  FaultSyn_efFaultSyn : Outport

== system DFADAS2_SenFus_v1_201204RC_training_210115/Signal Input (Input)/Signal Input (10ms) (Input10)/VehInfo/Vehicle Movement Signal Receive and Processing (VehMovRx)/Fault Synthesis (FaultSyn)2 ==
  in1 : Inport
  in2 : Inport  Port=2
  Constant : Constant  Value=0  OutDataTypeStr=uint16  SampleTime=-1
  FaultSyn_efFaultSyn : Outport
  wires:
  Constant/1 -> FaultSyn_efFaultSyn/1

== system DFADAS2_SenFus_v1_201204RC_training_210115/Signal Input (Input)/Signal Input (10ms) (Input10)/VehInfo/Vehicle Movement Signal Receive and Processing (VehMovRx)/VehLonAcc CAN Frame PreProcess (VehLonAccCANFrmPPrcs) ==
  CAN Unpack4 : canmsglib/CAN Unpack  CANdbFile=F:\LD\3_simulinkModel_13b\TJAHWA\ADAS_D53_PSA1CAN_LiPiao_DLC.dbc  MsgList=GW_32D_PSA1  MsgName=GW_32D_PSA1  MsgIDType=Standard (11-bit identifier)  MsgIdentifier=813  MsgLength=8  SignalInfo=ACCEL_LONGI_CALIB$12$12$2$2$1$0$2.000000e-02$-4.096000e+01$-4.096000e+01$4.092000e+01$#Brake_Pedal_Active$16$2$2$2$1$0$1$0$-Inf$Inf$#Braking_effort$9$1$2$2$1$0$1$0$-Inf$Inf$#ESC_ACC_Status$19$2$2$2$1$0$1$0$-Inf$Inf$#ESC_AEB_Status$10$2$2$2$1$0$1$0$-Inf$Inf$#Message_from_ESC_informing$23$1$2$2$1$0$1$0$-Inf$Inf$#UFC_to_ACC_dynamic_frame$56$4$2$2$1$0$1$0$-Inf$Inf$#Vehicle_Hold_Status$29$2$2$2$1$0$1$0$-Inf$Inf$#Vehicle_detected_as_stationary$21$1$2$2$1$0$1$0$-Inf$Inf$#YawRate_Raw$44$12$2$2$1$0$8.000000e-02$-1.638400e+02$-1.688400e+02$1.636800e+02$#bits_compute_counter_for_UCbrake$60$4$2$2$1$0$1$0$0$15$#  NSignals=11  IDPort=off  TimestampPort=off  ErrorPort=off  RemotePort=off  LengthPort=off  StatusPort=off  StartBits=str2num('[int32(12);int32(16);int32(9);int32(19);int32(10);int32(23);int32(56);int32(29);int32(21);int32(44);int32(60)]')  SignalSizes=str2num('[int32(12);int32(2);int32(1);int32(2);int32(2);int32(1);int32(4);int32(2);int32(1);int32(12);int32(4)]')  ByteOrders=str2num('[int32(2);int32(2);int32(2);int32(2);int32(2);int32(2);int32(2);int32(2);int32(2);int32(2);int32(2)]')  DataTypes=str2num('[int32(2);int32(2);int32(2);int32(2);int32(2);int32(2);int32(2);int32(2);int32(2);int32(2);int32(2)]')  MultiplexTypes=str2num('[int32(1);int32(1);int32(1);int32(1);int32(1);int32(1);int32(1);int32(1);int32(1);int32(1);int32(1)]')  MultiplexValues=str2num('[double(0);double(0);double(0);double(0);double(0);double(0);double(0);double(0);double(0);double(0);double(0)]')  Factors=str2num('[double(2.000000e-02);double(1);double(1);double(1);double(1);double(1);double(1);double(1);double(1);double(8.000000e-02);double(1)]')  Offsets=str2num('[double(-4.096000e+01);double(0);double(0);double(0);double(0);double(0);double(0);double(0);double(0);double(-1.638400e+02);double(0)]')  Minimums=str2num('[double(-4.096000e+01);double(-Inf);double(-Inf);double(-Inf);double(-Inf);double(-Inf);double(-Inf);double(-Inf);double(-Inf);double(-1.688400e+02);double(0)]')  Maximums=str2num('[double(4.092000e+01);double(Inf);double(Inf);double(Inf);double(Inf);double(Inf);double(Inf);double(Inf);double(Inf);double(1.636800e+02);double(15)]')  ApplyMinMax=off
      settings: SourceProductName=Simulink Real-Time  SourceProductBaseCode=XP  DataFormat=CANdb specified signals
  Data Type Conversion11 : DataTypeConversion  OutDataTypeStr=single
  Data Type Conversion{42,63..65} (4 alike) : DataTypeConversion  OutDataTypeStr=uint16
  Rate Transition{,1..4} (5 alike) : RateTransition  OutPortSampleTime=0.01
  S-Function1 : S-Function  FunctionName=NSTC297CANReceiveBlkLib  Parameters=|  SFunctionDeploymentMode=off  EnableBusSupport=off  mask(NSTC297 CAN Receive){Ns_DeviceID=ADAS Control Unit Gen2, Ns_ChannelNum=4, Ns_FrameID=813, Ns_IsVirtualFrame=off, Ns_RoleInVirtualFrame=Header Frame, Ns_HeaderFrameID=0, Ns_VirtualFrameStatusFlg=off, Ns_IncompleteFrameCntFlg=off, Ns_OverflowCntFlg=off, Ns_FrameBufferSize=1, Ns_SampleTime=0.02}
      | uint16(Ns_DeviceID),
      | uint16(Ns_ChannelNum),
      | uint32(Ns_FrameID),
      | uint8(Ns_IsVirtualFrame),
      | uint16(Ns_RoleInVirtualFrame),
      | uint32(Ns_HeaderFrameID),
      | uint8(Ns_VirtualFrameStatusFlg),
      | uint8(Ns_IncompleteFrameCntFlg),
      | uint8(Ns_OverflowCntFlg),
      | uint16(Ns_FrameBufferSize),
      | double(Ns_SampleTime)
      mask prompts: Ns_DeviceID "Device:"; Ns_ChannelNum "Channel number:"; Ns_FrameID "Frame ID:"; Ns_IsVirtualFrame "Belong to a virtual frame"; Ns_RoleInVirtualFrame "Position in virtual frame:"; Ns_HeaderFrameID "Header frame ID:"; Ns_VirtualFrameStatusFlg "Current virtural frame status output"; Ns_IncompleteFrameCntFlg "Incomplete virtual frame count output"; Ns_OverflowCntFlg "Overflow count output"; Ns_FrameBufferSize "Frame buffer size:"; Ns_SampleTime "Sample time:"
      mask init:
      | NSTC297CANReceive_callback('portlabels');
      mask TypeOptions Ns_DeviceID: General Control Unit Gen2 | ADAS Control Unit Gen2
      mask TypeOptions Ns_ChannelNum: 0 | 1 | 2 | 3 | 4 | 5
      mask Callback Ns_IsVirtualFrame: NSTC297CANReceive_callback('Belong to a virtual frame');
      mask TypeOptions Ns_RoleInVirtualFrame: Header Frame | Data Frame | Trailer Frame
      mask Callback Ns_RoleInVirtualFrame: NSTC297CANReceive_callback('Position in virtual frame');
      mask Display: color('blue');text(0.02,0.9,'NovSteeds TC297','horizontalAlignment','left');color('blue');text(0.5,0.7,'CAN Receive','horizontalAlignment','center');color('black');text(0.5,0.6,'Channel: 4','horizontalAlignment','center');text(0.5,0.5,'ID: 813','horizontalAlignment','center');text(0.5,0.4,'Virtual Frame: No','horizontalAlignment','center');port_label('output',1, 'RemainderCnt');port_label('output',2, 'Msg');
  ESC_LongitudinalAcc : Outport
  ESC_ACC_Status : Outport  Port=2
  ESC_AEB_Status : Outport  Port=3
  Message_from_ESC_informing : Outport  Port=4
  Vehicle_detected_as_stationary : Outport  Port=5
  wires:
  S-Function1/2 -> CAN Unpack4/1
  Data Type Conversion11/1 -> ESC_LongitudinalAcc/1  "ESC_LongitudinalAcc"
  CAN Unpack4/1 -> Rate Transition/1
  Rate Transition/1 -> Data Type Conversion11/1
  Data Type Conversion65/1 -> ESC_ACC_Status/1
  Data Type Conversion63/1 -> Message_from_ESC_informing/1
  Data Type Conversion64/1 -> ESC_AEB_Status/1
  Data Type Conversion42/1 -> Vehicle_detected_as_stationary/1
  CAN Unpack4/9 -> Rate Transition4/1
  CAN Unpack4/6 -> Rate Transition3/1
  CAN Unpack4/5 -> Rate Transition2/1
  CAN Unpack4/4 -> Rate Transition1/1
  Rate Transition1/1 -> Data Type Conversion65/1
  Rate Transition2/1 -> Data Type Conversion64/1
  Rate Transition3/1 -> Data Type Conversion63/1
  Rate Transition4/1 -> Data Type Conversion42/1

== system DFADAS2_SenFus_v1_201204RC_training_210115/Signal Input (Input)/Signal Input (10ms) (Input10)/VehInfo/Vehicle Movement Signal Receive and Processing (VehMovRx)/VehSpd CAN Frame PreProcess (VehSpdCANFrmPPrcs) ==
  CAN Diagnosis (CANDia) : Subsystem  Commented=on
  CAN Receive Sample Time : Constant  Value=0.02  OutDataTypeStr=single  SampleTime=-1
  CAN Unpack : canmsglib/CAN Unpack  CANdbFile=F:\LD\3_simulinkModel_13b\TJAHWA\ADAS_D53_PSA1CAN_LiPiao_DLC.dbc  MsgList=ESC_38D_PSA1  MsgName=ESC_38D_PSA1  MsgIDType=Standard (11-bit identifier)  MsgIdentifier=909  MsgLength=8  SignalInfo=ABR_dynamic_checksum$40$4$2$2$1$0$1$0$-Inf$Inf$#Vehicle_driving_direction$52$2$2$2$1$0$1$0$-Inf$Inf$#Vehicle_speed_of_wheelsensor$8$16$2$2$1$0$1.000000e-02$0$0$6.553400e+02$#Vehiclespeed_unavailability_flag$50$2$2$2$1$0$1$0$-Inf$Inf$#bits_compute_for_UC_brake$44$4$2$2$1$0$1$0$0$15$#  NSignals=5  IDPort=off  TimestampPort=off  ErrorPort=off  RemotePort=off  LengthPort=off  StatusPort=off  StartBits=str2num('[int32(40);int32(52);int32(8);int32(50);int32(44)]')  SignalSizes=str2num('[int32(4);int32(2);int32(16);int32(2);int32(4)]')  ByteOrders=str2num('[int32(2);int32(2);int32(2);int32(2);int32(2)]')  DataTypes=str2num('[int32(2);int32(2);int32(2);int32(2);int32(2)]')  MultiplexTypes=str2num('[int32(1);int32(1);int32(1);int32(1);int32(1)]')  MultiplexValues=str2num('[double(0);double(0);double(0);double(0);double(0)]')  Factors=str2num('[double(1);double(1);double(1.000000e-02);double(1);double(1)]')  Offsets=str2num('[double(0);double(0);double(0);double(0);double(0)]')  Minimums=str2num('[double(-Inf);double(-Inf);double(0);double(-Inf);double(0)]')  Maximums=str2num('[double(Inf);double(Inf);double(6.553400e+02);double(Inf);double(15)]')  ApplyMinMax=off
      settings: SourceProductName=Simulink Real-Time  SourceProductBaseCode=XP  DataFormat=CANdb specified signals
  Constant : Constant  Value=0  OutDataTypeStr=single
  Data Type Conversion{1,3,5..7} (5 alike) : DataTypeConversion  OutDataTypeStr=single
  Data Type Conversion53 : DataTypeConversion  OutDataTypeStr=uint16
  Data Type Conversion82 : DataTypeConversion  OutDataTypeStr=uint16
  Rate Transition{1..7} (7 alike) : RateTransition  OutPortSampleTime=0.01
  S-Function1 : S-Function  FunctionName=NSTC297CANReceiveBlkLib  Parameters=|  SFunctionDeploymentMode=off  EnableBusSupport=off  mask(NSTC297 CAN Receive){Ns_DeviceID=ADAS Control Unit Gen2, Ns_ChannelNum=4, Ns_FrameID=909, Ns_IsVirtualFrame=off, Ns_RoleInVirtualFrame=Header Frame, Ns_HeaderFrameID=0, Ns_VirtualFrameStatusFlg=off, Ns_IncompleteFrameCntFlg=off, Ns_OverflowCntFlg=off, Ns_FrameBufferSize=1, Ns_SampleTime=0.04}
      | uint16(Ns_DeviceID),
      | uint16(Ns_ChannelNum),
      | uint32(Ns_FrameID),
      | uint8(Ns_IsVirtualFrame),
      | uint16(Ns_RoleInVirtualFrame),
      | uint32(Ns_HeaderFrameID),
      | uint8(Ns_VirtualFrameStatusFlg),
      | uint8(Ns_IncompleteFrameCntFlg),
      | uint8(Ns_OverflowCntFlg),
      | uint16(Ns_FrameBufferSize),
      | double(Ns_SampleTime)
      mask prompts: Ns_DeviceID "Device:"; Ns_ChannelNum "Channel number:"; Ns_FrameID "Frame ID:"; Ns_IsVirtualFrame "Belong to a virtual frame"; Ns_RoleInVirtualFrame "Position in virtual frame:"; Ns_HeaderFrameID "Header frame ID:"; Ns_VirtualFrameStatusFlg "Current virtural frame status output"; Ns_IncompleteFrameCntFlg "Incomplete virtual frame count output"; Ns_OverflowCntFlg "Overflow count output"; Ns_FrameBufferSize "Frame buffer size:"; Ns_SampleTime "Sample time:"
      mask init:
      | NSTC297CANReceive_callback('portlabels');
      mask TypeOptions Ns_DeviceID: General Control Unit Gen2 | ADAS Control Unit Gen2
      mask TypeOptions Ns_ChannelNum: 0 | 1 | 2 | 3 | 4 | 5
      mask Callback Ns_IsVirtualFrame: NSTC297CANReceive_callback('Belong to a virtual frame');
      mask TypeOptions Ns_RoleInVirtualFrame: Header Frame | Data Frame | Trailer Frame
      mask Callback Ns_RoleInVirtualFrame: NSTC297CANReceive_callback('Position in virtual frame');
      mask Display: color('blue');text(0.02,0.9,'NovSteeds TC297','horizontalAlignment','left');color('blue');text(0.5,0.7,'CAN Receive','horizontalAlignment','center');color('black');text(0.5,0.6,'Channel: 4','horizontalAlignment','center');text(0.5,0.5,'ID: 909','horizontalAlignment','center');text(0.5,0.4,'Virtual Frame: No','horizontalAlignment','center');port_label('output',1, 'RemainderCnt');port_label('output',2, 'Msg');
  Time Limit : Constant  OutDataTypeStr=single  SampleTime=-1
  Out1 : Outport
  Vehicle_driving_direction : Outport  Port=2
  out : Outport  Port=3
  Vehiclespeed_unavailability_flag : Outport  Port=4
  CANFrmPPrcs_vVehSpd : Outport  Port=5
  Out6 : Outport  Port=6
  Out7 : Outport  Port=7
  wires:
  CAN Receive Sample Time/1 -> CAN Diagnosis (CANDia)/1(CANDia_tiCANRxSmplT)
  Time Limit/1 -> CAN Diagnosis (CANDia)/2(CANDia_tiTLim)
  S-Function1/1 -> CAN Diagnosis (CANDia)/3(CANDia_cfNewFlg)
  S-Function1/2 -> CAN Diagnosis (CANDia)/4(CANDia_regCANMsg), CAN Unpack/1
  Rate Transition1/1 -> Data Type Conversion1/1
  Rate Transition2/1 -> Data Type Conversion53/1
  Rate Transition4/1 -> Data Type Conversion82/1
  Rate Transition5/1 -> Data Type Conversion5/1
  Rate Transition6/1 -> Data Type Conversion6/1
  Rate Transition7/1 -> Data Type Conversion7/1
  Data Type Conversion1/1 -> Out1/1
  Data Type Conversion5/1 -> CANFrmPPrcs_vVehSpd/1
  Data Type Conversion6/1 -> Out6/1
  Data Type Conversion7/1 -> Out7/1
  CAN Unpack/3 -> Rate Transition5/1
  Rate Transition3/1 -> Data Type Conversion3/1
  Data Type Conversion3/1 -> out/1
  Constant/1 -> Rate Transition3/1
  Data Type Conversion53/1 -> Vehiclespeed_unavailability_flag/1
  Data Type Conversion82/1 -> Vehicle_driving_direction/1
  CAN Unpack/2 -> Rate Transition4/1
  CAN Unpack/4 -> Rate Transition2/1
